simulink model "HVAC_Distribuito"  (R2025a)
settings: Solver=VariableStepAuto  StartTime=0.0  StopTime=10000  RelTol=1e-3
undefined symbols (not defined in the file): C, epsilon, Err_thr, Kd, Ki, Kp, L, P_max, P_max_high, P_max_low, R, T_ext, T_setpoint_desiderati
libraries: slpidlib x3, simulink x3
settings Model: Creator=smant  LastModifiedBy=smant

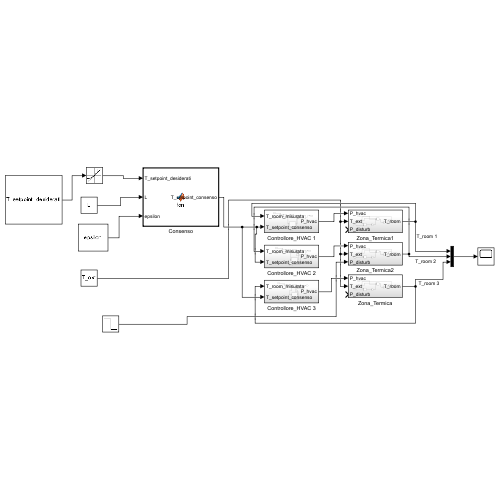
[thumbnail: Simulink's stored preview of the top-level diagram]
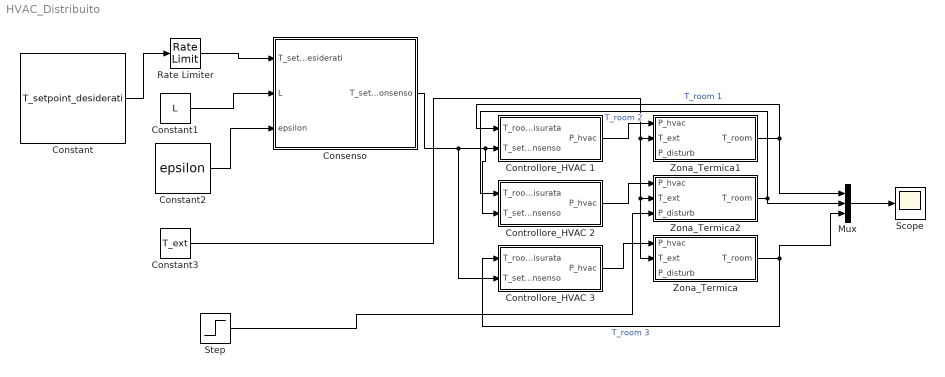
== system HVAC_Distribuito ==
  Consenso : MATLAB Function  TreatAsAtomicUnit=on
  Constant : Constant  Value=T_setpoint_desiderati
  Constant1 : Constant  Value=L
  Constant2 : Constant  Value=epsilon
  Constant3 : Constant  Value=T_ext
  Controllore_HVAC 1 : Subsystem
  Controllore_HVAC 2 : Subsystem
  Controllore_HVAC 3 : Subsystem
  Mux : Mux  Inputs=3
  Rate Limiter : RateLimiter  RisingSlewLimit=0.032  FallingSlewLimit=-0.01  SampleTimeMode=inherited  InitialCondition=5
  Scope : Scope
      settings: ActiveDisplayYMinimum=-9.9704836067094789  ActiveDisplayYMaximum=45.777608199234592
  Step : Step  Time=1800  After=-500  SampleTime=0
  Zona_Termica : Subsystem
  Zona_Termica1 : Subsystem
  Zona_Termica2 : Subsystem
  wires:
  Constant2/1 -> Consenso/3(epsilon)
  Constant1/1 -> Consenso/2(L)
  Controllore_HVAC 1/1(P_hvac) -> Zona_Termica1/1(P_hvac)
  Zona_Termica1/1(T_room) -> Mux/1, Controllore_HVAC 1/1(T_room_misurata)  "T_room 1"
  Controllore_HVAC 2/1(P_hvac) -> Zona_Termica2/1(P_hvac)
  Zona_Termica2/1(T_room) -> Mux/2, Controllore_HVAC 2/1(T_room_misurata)  "T_room 2"
  Controllore_HVAC 3/1(P_hvac) -> Zona_Termica/1(P_hvac)
  Zona_Termica/1(T_room) -> Mux/3, Controllore_HVAC 3/1(T_room_misurata)  "T_room 3"
  Constant3/1 -> Zona_Termica2/2(T_ext), Zona_Termica/2(T_ext), Zona_Termica1/2(T_ext)
  Step/1 -> Zona_Termica2/3(P_disturb)
  Mux/1 -> Scope/1
  Consenso/1(T_setpoint_consenso) -> Controllore_HVAC 2/2(T_setpoint_consenso), Controllore_HVAC 1/2(T_setpoint_consenso), Controllore_HVAC 3/2(T_setpoint_consenso)
  Constant/1 -> Rate Limiter/1
  Rate Limiter/1 -> Consenso/1(T_setpoint_desiderati)

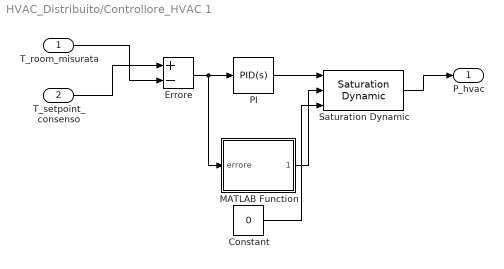
== system HVAC_Distribuito/Controllore_HVAC 1 ==
  T_room_misurata : Inport
  T_setpoint_consenso : Inport  Port=2
  Constant : Constant  Value=0
  Errore : Sum  Inputs=+-
  MATLAB Function : MATLAB Function  TreatAsAtomicUnit=on
  PI : slpidlib/PID Controller  Controller=PID  Form=Parallel  TimeDomain=Continuous-time  UseExternalTs=off  SampleTime=-1  IntegratorMethod=Forward Euler  FilterMethod=Forward Euler  ControllerParametersSource=internal  P=Kp  I=Ki  UseKiTs=off  D=Kd  UseExternalDerivativeSource=off  N=10  UseFilter=on  TunerSelectOption=Transfer Function Based (PID Tuner App)  InitialConditionSource=internal  InitialConditionForIntegrator=0  InitialConditionForFilter=0  DifferentiatorICPrevScaledInput=0  ExternalReset=none  TrackingMode=off  Kt=1  LimitOutput=off  SatLimitsSource=internal  UpperSaturationLimit=P_max  LowerSaturationLimit=0  LinearizeAsGain=on  AntiWindupMode=clamping  Kb=1  LimitIntegrator=off  UpperIntegratorSaturationLimit=inf  LowerIntegratorSaturationLimit=-inf  POutMin=[]  POutMax=[]  IOutMin=[]  IOutMax=[]  DOutMin=[]  DOutMax=[]  NOutMin=[]  NOutMax=[]  SumOutMin=[]  SumOutMax=[]  SaturationOutMin=[]  SaturationOutMax=[]  PParamMin=[]  PParamMax=[]  IParamMin=[]  IParamMax=[]  DParamMin=[]  DParamMax=[]  NParamMin=[]  NParamMax=[]  KbParamMin=[]  KbParamMax=[]  KtParamMin=[]  KtParamMax=[]  KbOutMin=[]  KbOutMax=[]  KtOutMin=[]  KtOutMax=[]  IntegratorOutMin=[]  IntegratorOutMax=[]  FilterOutMin=[]  FilterOutMax=[]  SumI1OutMin=[]  SumI1OutMax=[]  SumI2OutMin=[]  SumI2OutMax=[]  SumI3OutMin=[]  SumI3OutMax=[]  SumI4OutMin=[]  SumI4OutMax=[]  SumDOutMin=[]  SumDOutMax=[]  DifferentiatorOutMin=[]  DifferentiatorOutMax=[]  FilterDiffOutCoefMin=[]  FilterDiffOutCoefMax=[]  ReciprocalOutMin=[]  ReciprocalOutMax=[]  SumDenOutMin=[]  SumDenOutMax=[]  SumNumOutMin=[]  SumNumOutMax=[]  DivideOutMin=[]  DivideOutMax=[]  UdiffTsProdOutMin=[]  UdiffTsProdOutMax=[]  NTsProdOutMin=[]  NTsProdOutMax=[]  UintegralTsProdOutMin=[]  UintegralTsProdOutMax=[]  UngainTsProdOutMin=[]  UngainTsProdOutMax=[]  ClampingZeroOutDataTypeStr=Inherit: Inherit via back propagation  ClampingZeroOutMin=[]  ClampingZeroOutMax=[]  FilterDenConstantOutDataTypeStr=Inherit: Inherit via back propagation  FilterDenConstantOutMin=[]  FilterDenConstantOutMax=[]  PCopyOutDataTypeStr=Inherit: Inherit via back propagation  PCopyOutMin=[]  PCopyOutMax=[]  NCopyOutDataTypeStr=Inherit: Inherit via back propagation  NCopyOutMin=[]  NCopyOutMax=[]  IntegratorContinuousStateAttributes=''  IntegratorStateMustResolveToSignalObject=off  IntegratorRTWStateStorageClass=Auto  FilterContinuousStateAttributes=''  FilterStateMustResolveToSignalObject=off  FilterRTWStateStorageClass=Auto  ParallelPVariant=InternalParameters  IdealPVariant=Disabled  IVariant=InternalParameters  DVariant=InternalParameters  IntegratorVariant=Continuous  SatVariant=Disabled  AWVariant=Passthrough  PCopyVariant=Disabled  TRVariant=Disabled  FdbkBlocksVariant=Forward  IdealPFdbkVariant=Disabled  SatFdbkVariant=Disabled  DerivativeFilterVariant=ContFilter  NVariant=InternalParameters  NCopyVariant=Disabled  FilterICVariant=InternalICsFilter  IntegratorICVariant=InternalICs  ExternalResetVariant=Disabled  TRSumVariant=Passthrough  SumFdbkVariant=Disabled  SumVariant=Sum_PID  TsampFilterVariant=InternalTs  TsampNgainVariant=Passthrough  TsampIntegralVariant=Disabled_SignalSpec  ExternalSaturationOutDataTypeStr=Inherit: Same as second input  DerivativeSourceVariant=ErrorSignal  PreIntVariant=InternalPreInt
  Saturation Dynamic : simulink/Discontinuities/Saturation Dynamic  OutMin=[]  OutMax=[]  OutDataTypeStr=Inherit: Same as second input  OutDataType=fixdt(1, 16)  OutScaling=2^-10  DoSatur=off
  P_hvac : Outport
  wires:
  T_room_misurata/1 -> Errore/2
  T_setpoint_consenso/1 -> Errore/1
  Errore/1 -> MATLAB Function/1(errore), PI/1
  Saturation Dynamic/1 -> P_hvac/1
  PI/1 -> Saturation Dynamic/1
  MATLAB Function/1(P_max_dinamico) -> Saturation Dynamic/2
  Constant/1 -> Saturation Dynamic/3

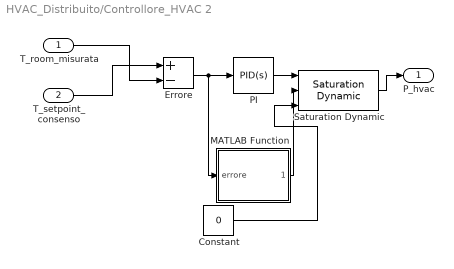
== system HVAC_Distribuito/Controllore_HVAC 2 ==
  T_room_misurata : Inport
  T_setpoint_consenso : Inport  Port=2
  Constant : Constant  Value=0
  Errore : Sum  Inputs=+-
  MATLAB Function : MATLAB Function  TreatAsAtomicUnit=on
  PI : slpidlib/PID Controller  Controller=PID  Form=Parallel  TimeDomain=Continuous-time  UseExternalTs=off  SampleTime=-1  IntegratorMethod=Forward Euler  FilterMethod=Forward Euler  ControllerParametersSource=internal  P=Kp  I=Ki  UseKiTs=off  D=Kd  UseExternalDerivativeSource=off  N=10  UseFilter=on  TunerSelectOption=Transfer Function Based (PID Tuner App)  InitialConditionSource=internal  InitialConditionForIntegrator=0  InitialConditionForFilter=0  DifferentiatorICPrevScaledInput=0  ExternalReset=none  TrackingMode=off  Kt=1  LimitOutput=off  SatLimitsSource=internal  UpperSaturationLimit=P_max  LowerSaturationLimit=0  LinearizeAsGain=on  AntiWindupMode=clamping  Kb=1  LimitIntegrator=off  UpperIntegratorSaturationLimit=inf  LowerIntegratorSaturationLimit=-inf  POutMin=[]  POutMax=[]  IOutMin=[]  IOutMax=[]  DOutMin=[]  DOutMax=[]  NOutMin=[]  NOutMax=[]  SumOutMin=[]  SumOutMax=[]  SaturationOutMin=[]  SaturationOutMax=[]  PParamMin=[]  PParamMax=[]  IParamMin=[]  IParamMax=[]  DParamMin=[]  DParamMax=[]  NParamMin=[]  NParamMax=[]  KbParamMin=[]  KbParamMax=[]  KtParamMin=[]  KtParamMax=[]  KbOutMin=[]  KbOutMax=[]  KtOutMin=[]  KtOutMax=[]  IntegratorOutMin=[]  IntegratorOutMax=[]  FilterOutMin=[]  FilterOutMax=[]  SumI1OutMin=[]  SumI1OutMax=[]  SumI2OutMin=[]  SumI2OutMax=[]  SumI3OutMin=[]  SumI3OutMax=[]  SumI4OutMin=[]  SumI4OutMax=[]  SumDOutMin=[]  SumDOutMax=[]  DifferentiatorOutMin=[]  DifferentiatorOutMax=[]  FilterDiffOutCoefMin=[]  FilterDiffOutCoefMax=[]  ReciprocalOutMin=[]  ReciprocalOutMax=[]  SumDenOutMin=[]  SumDenOutMax=[]  SumNumOutMin=[]  SumNumOutMax=[]  DivideOutMin=[]  DivideOutMax=[]  UdiffTsProdOutMin=[]  UdiffTsProdOutMax=[]  NTsProdOutMin=[]  NTsProdOutMax=[]  UintegralTsProdOutMin=[]  UintegralTsProdOutMax=[]  UngainTsProdOutMin=[]  UngainTsProdOutMax=[]  ClampingZeroOutDataTypeStr=Inherit: Inherit via back propagation  ClampingZeroOutMin=[]  ClampingZeroOutMax=[]  FilterDenConstantOutDataTypeStr=Inherit: Inherit via back propagation  FilterDenConstantOutMin=[]  FilterDenConstantOutMax=[]  PCopyOutDataTypeStr=Inherit: Inherit via back propagation  PCopyOutMin=[]  PCopyOutMax=[]  NCopyOutDataTypeStr=Inherit: Inherit via back propagation  NCopyOutMin=[]  NCopyOutMax=[]  IntegratorContinuousStateAttributes=''  IntegratorStateMustResolveToSignalObject=off  IntegratorRTWStateStorageClass=Auto  FilterContinuousStateAttributes=''  FilterStateMustResolveToSignalObject=off  FilterRTWStateStorageClass=Auto  ParallelPVariant=InternalParameters  IdealPVariant=Disabled  IVariant=InternalParameters  DVariant=InternalParameters  IntegratorVariant=Continuous  SatVariant=Disabled  AWVariant=Passthrough  PCopyVariant=Disabled  TRVariant=Disabled  FdbkBlocksVariant=Forward  IdealPFdbkVariant=Disabled  SatFdbkVariant=Disabled  DerivativeFilterVariant=ContFilter  NVariant=InternalParameters  NCopyVariant=Disabled  FilterICVariant=InternalICsFilter  IntegratorICVariant=InternalICs  ExternalResetVariant=Disabled  TRSumVariant=Passthrough  SumFdbkVariant=Disabled  SumVariant=Sum_PID  TsampFilterVariant=InternalTs  TsampNgainVariant=Passthrough  TsampIntegralVariant=Disabled_SignalSpec  ExternalSaturationOutDataTypeStr=Inherit: Same as second input  DerivativeSourceVariant=ErrorSignal  PreIntVariant=InternalPreInt
  Saturation Dynamic : simulink/Discontinuities/Saturation Dynamic  OutMin=[]  OutMax=[]  OutDataTypeStr=Inherit: Same as second input  OutDataType=fixdt(1, 16)  OutScaling=2^-10  DoSatur=off
  P_hvac : Outport
  wires:
  T_room_misurata/1 -> Errore/2
  T_setpoint_consenso/1 -> Errore/1
  Errore/1 -> MATLAB Function/1(errore), PI/1
  PI/1 -> Saturation Dynamic/1
  Saturation Dynamic/1 -> P_hvac/1
  MATLAB Function/1(P_max_dinamico) -> Saturation Dynamic/2
  Constant/1 -> Saturation Dynamic/3

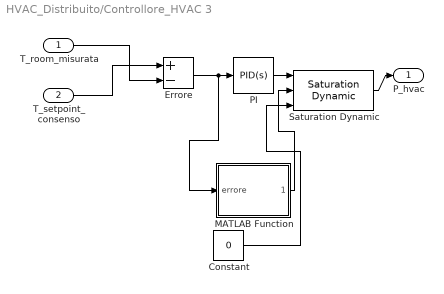
== system HVAC_Distribuito/Controllore_HVAC 3 ==
  T_room_misurata : Inport
  T_setpoint_consenso : Inport  Port=2
  Constant : Constant  Value=0
  Errore : Sum  Inputs=+-
  MATLAB Function : MATLAB Function  TreatAsAtomicUnit=on
  PI : slpidlib/PID Controller  Controller=PID  Form=Parallel  TimeDomain=Continuous-time  UseExternalTs=off  SampleTime=-1  IntegratorMethod=Forward Euler  FilterMethod=Forward Euler  ControllerParametersSource=internal  P=Kp  I=Ki  UseKiTs=off  D=Kd  UseExternalDerivativeSource=off  N=10  UseFilter=on  TunerSelectOption=Transfer Function Based (PID Tuner App)  InitialConditionSource=internal  InitialConditionForIntegrator=0  InitialConditionForFilter=0  DifferentiatorICPrevScaledInput=0  ExternalReset=none  TrackingMode=off  Kt=1  LimitOutput=on  SatLimitsSource=internal  UpperSaturationLimit=P_max  LowerSaturationLimit=0  LinearizeAsGain=on  AntiWindupMode=clamping  Kb=1  LimitIntegrator=off  UpperIntegratorSaturationLimit=inf  LowerIntegratorSaturationLimit=-inf  POutMin=[]  POutMax=[]  IOutMin=[]  IOutMax=[]  DOutMin=[]  DOutMax=[]  NOutMin=[]  NOutMax=[]  SumOutMin=[]  SumOutMax=[]  SaturationOutMin=[]  SaturationOutMax=[]  PParamMin=[]  PParamMax=[]  IParamMin=[]  IParamMax=[]  DParamMin=[]  DParamMax=[]  NParamMin=[]  NParamMax=[]  KbParamMin=[]  KbParamMax=[]  KtParamMin=[]  KtParamMax=[]  KbOutMin=[]  KbOutMax=[]  KtOutMin=[]  KtOutMax=[]  IntegratorOutMin=[]  IntegratorOutMax=[]  FilterOutMin=[]  FilterOutMax=[]  SumI1OutMin=[]  SumI1OutMax=[]  SumI2OutMin=[]  SumI2OutMax=[]  SumI3OutMin=[]  SumI3OutMax=[]  SumI4OutMin=[]  SumI4OutMax=[]  SumDOutMin=[]  SumDOutMax=[]  DifferentiatorOutMin=[]  DifferentiatorOutMax=[]  FilterDiffOutCoefMin=[]  FilterDiffOutCoefMax=[]  ReciprocalOutMin=[]  ReciprocalOutMax=[]  SumDenOutMin=[]  SumDenOutMax=[]  SumNumOutMin=[]  SumNumOutMax=[]  DivideOutMin=[]  DivideOutMax=[]  UdiffTsProdOutMin=[]  UdiffTsProdOutMax=[]  NTsProdOutMin=[]  NTsProdOutMax=[]  UintegralTsProdOutMin=[]  UintegralTsProdOutMax=[]  UngainTsProdOutMin=[]  UngainTsProdOutMax=[]  ClampingZeroOutDataTypeStr=Inherit: Inherit via back propagation  ClampingZeroOutMin=[]  ClampingZeroOutMax=[]  FilterDenConstantOutDataTypeStr=Inherit: Inherit via back propagation  FilterDenConstantOutMin=[]  FilterDenConstantOutMax=[]  PCopyOutDataTypeStr=Inherit: Inherit via back propagation  PCopyOutMin=[]  PCopyOutMax=[]  NCopyOutDataTypeStr=Inherit: Inherit via back propagation  NCopyOutMin=[]  NCopyOutMax=[]  IntegratorContinuousStateAttributes=''  IntegratorStateMustResolveToSignalObject=off  IntegratorRTWStateStorageClass=Auto  FilterContinuousStateAttributes=''  FilterStateMustResolveToSignalObject=off  FilterRTWStateStorageClass=Auto  ParallelPVariant=InternalParameters  IdealPVariant=Disabled  IVariant=InternalParameters  DVariant=InternalParameters  IntegratorVariant=Continuous  SatVariant=Enabled  AWVariant=ContClampingParallel  PCopyVariant=Disabled  TRVariant=Disabled  FdbkBlocksVariant=Forward  IdealPFdbkVariant=Disabled  SatFdbkVariant=Disabled  DerivativeFilterVariant=ContFilter  NVariant=InternalParameters  NCopyVariant=Disabled  FilterICVariant=InternalICsFilter  IntegratorICVariant=InternalICs  ExternalResetVariant=Disabled  TRSumVariant=Passthrough  SumFdbkVariant=Disabled  SumVariant=Sum_PID  TsampFilterVariant=InternalTs  TsampNgainVariant=Passthrough  TsampIntegralVariant=Disabled_SignalSpec  ExternalSaturationOutDataTypeStr=Inherit: Same as second input  DerivativeSourceVariant=ErrorSignal  PreIntVariant=InternalPreInt
  Saturation Dynamic : simulink/Discontinuities/Saturation Dynamic  OutMin=[]  OutMax=[]  OutDataTypeStr=Inherit: Same as second input  OutDataType=fixdt(1, 16)  OutScaling=2^-10  DoSatur=off
  P_hvac : Outport
  wires:
  T_room_misurata/1 -> Errore/2
  T_setpoint_consenso/1 -> Errore/1
  Errore/1 -> MATLAB Function/1(errore), PI/1
  PI/1 -> Saturation Dynamic/1
  Saturation Dynamic/1 -> P_hvac/1
  MATLAB Function/1(P_max_dinamico) -> Saturation Dynamic/2
  Constant/1 -> Saturation Dynamic/3

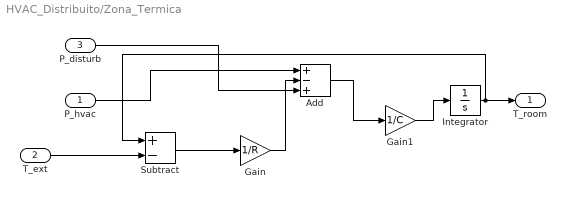
== system HVAC_Distribuito/Zona_Termica ==
  P_hvac : Inport
  T_ext : Inport  Port=2
  P_disturb : Inport  Port=3
  Add : Sum  Inputs=+-+
  Gain : Gain  Gain=1/R
  Gain1 : Gain  Gain=1/C
  Integrator : Integrator  InitialCondition=T_ext  LimitOutput=on  UpperSaturationLimit=30
  Subtract : Sum  Inputs=+-
  T_room : Outport
  wires:
  T_ext/1 -> Subtract/2
  Subtract/1 -> Gain/1
  P_hvac/1 -> Add/1
  Gain/1 -> Add/2
  P_disturb/1 -> Add/3
  Add/1 -> Gain1/1
  Gain1/1 -> Integrator/1
  Integrator/1 -> Subtract/1, T_room/1

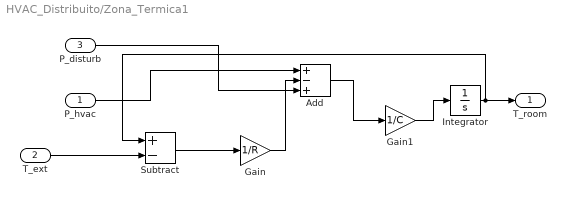
== system HVAC_Distribuito/Zona_Termica1 ==
  P_hvac : Inport
  T_ext : Inport  Port=2
  P_disturb : Inport  Port=3
  Add : Sum  Inputs=+-+
  Gain : Gain  Gain=1/R
  Gain1 : Gain  Gain=1/C
  Integrator : Integrator  InitialCondition=T_ext  LimitOutput=on  UpperSaturationLimit=30
  Subtract : Sum  Inputs=+-
  T_room : Outport
  wires:
  T_ext/1 -> Subtract/2
  Subtract/1 -> Gain/1
  P_hvac/1 -> Add/1
  Gain/1 -> Add/2
  P_disturb/1 -> Add/3
  Add/1 -> Gain1/1
  Gain1/1 -> Integrator/1
  Integrator/1 -> Subtract/1, T_room/1

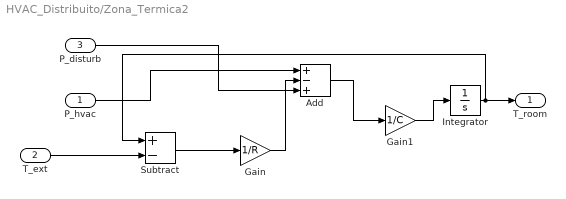
== system HVAC_Distribuito/Zona_Termica2 ==
  P_hvac : Inport
  T_ext : Inport  Port=2
  P_disturb : Inport  Port=3
  Add : Sum  Inputs=+-+
  Gain : Gain  Gain=1/R
  Gain1 : Gain  Gain=1/C
  Integrator : Integrator  InitialCondition=T_ext  LimitOutput=on  UpperSaturationLimit=30
  Subtract : Sum  Inputs=+-
  T_room : Outport
  wires:
  T_ext/1 -> Subtract/2
  Subtract/1 -> Gain/1
  P_hvac/1 -> Add/1
  Gain/1 -> Add/2
  P_disturb/1 -> Add/3
  Add/1 -> Gain1/1
  Gain1/1 -> Integrator/1
  Integrator/1 -> Subtract/1, T_room/1

== matlab function HVAC_Distribuito/Controllore_HVAC 1/MATLAB Function ==
  data: errore input; P_max_dinamico output; P_max_high parameter; P_max_low parameter; Err_thr parameter
function P_max_dinamico = fcn(errore, P_max_high, P_max_low, Err_thr)
%#codegen
% Questa funzione riceve l'errore e i parametri,
% e restituisce il limite di potenza corretto.

if abs(errore) > Err_thr
    % Errore grande (Avvio): usa la potenza "soft"
    P_max_dinamico = P_max_low;
else
    % Errore piccolo (Controllo): usa la potenza massima
    P_max_dinamico = P_max_high;
end

== matlab function HVAC_Distribuito/Consenso ==
  data: T_setpoint_desiderati input; T_setpoint_consenso output; L input; epsilon input
function T_setpoint_consenso = fcn(T_setpoint_desiderati, L, epsilon)

    % Dichiara la variabile di stato (persistente)
    % Questa variabile mantiene il suo valore tra le esecuzioni
    persistent x; 

    % Inizializza lo stato al primo ciclo
    if isempty(x)
        x = T_setpoint_desiderati;
    end

    % Algoritmo di Consenso Lineare (Average Consensus in tempo continuo)
    % dx/dt = -L * x
    % Lo discretizziamo: x(k+1) = x(k) - epsilon * L * x(k)

    % Calcola il passo di consenso
    x_dot = -L * x;

    % Aggiorna lo stato usando Eulero (semplice discretizzazione)
    % Nota: 'epsilon' qui funge da nostro "passo di integrazione" dt
    x = x + epsilon * x_dot; 

    % L'output è lo stato attuale dei setpoint
    T_setpoint_consenso = x;

end

== matlab function HVAC_Distribuito/Controllore_HVAC 2/MATLAB Function ==
  data: errore input; P_max_dinamico output; P_max_high parameter; P_max_low parameter; Err_thr parameter
function P_max_dinamico = fcn(errore, P_max_high, P_max_low, Err_thr)
%#codegen
% Questa funzione riceve l'errore e i parametri,
% e restituisce il limite di potenza corretto.

if abs(errore) > Err_thr
    % Errore grande (Avvio): usa la potenza "soft"
    P_max_dinamico = P_max_low;
else
    % Errore piccolo (Controllo): usa la potenza massima
    P_max_dinamico = P_max_high;
end

== matlab function HVAC_Distribuito/Controllore_HVAC 3/MATLAB Function ==
  data: errore input; P_max_dinamico output; P_max_high parameter; P_max_low parameter; Err_thr parameter
function P_max_dinamico = fcn(errore, P_max_high, P_max_low, Err_thr)
%#codegen
% Questa funzione riceve l'errore e i parametri,
% e restituisce il limite di potenza corretto.

if abs(errore) > Err_thr
    % Errore grande (Avvio): usa la potenza "soft"
    P_max_dinamico = P_max_low;
else
    % Errore piccolo (Controllo): usa la potenza massima
    P_max_dinamico = P_max_high;
end
